simulink model "Q2_C_D_E"  (R2021a)
settings: Solver=VariableStepAuto  StartTime=0.0  StopTime=1  RelTol=1e-3
settings Model: Creator=Mohammad  LastModifiedBy=Mohammad

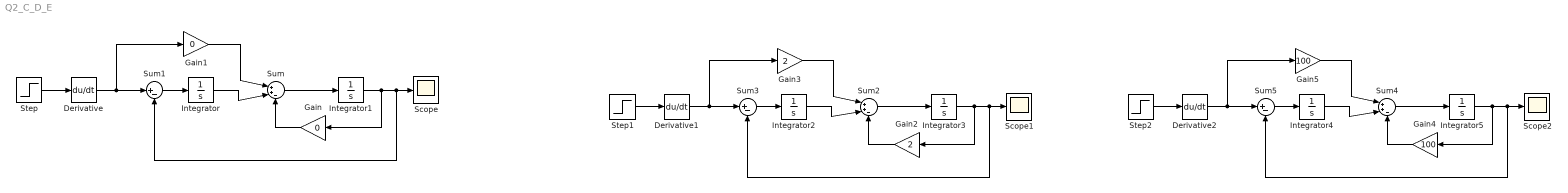
== system Q2_C_D_E ==
  Derivative : Derivative
  Derivative1 : Derivative
  Derivative2 : Derivative
  Gain : Gain  Gain=0
  Gain1 : Gain  Gain=0
  Gain2 : Gain  Gain=2
  Gain3 : Gain  Gain=2
  Gain4 : Gain  Gain=100
  Gain5 : Gain  Gain=100
  Integrator{,1..5} (6 alike) : Integrator
  Scope : Scope
  Scope1 : Scope
  Scope2 : Scope
  Step : Step  Time=0.001  SampleTime=0
  Step1 : Step  Time=0.001  SampleTime=0
  Step2 : Step  Time=0.001  SampleTime=0
  Sum : Sum  Inputs=|++-
  Sum1 : Sum  Inputs=|+-
  Sum2 : Sum  Inputs=|++-
  Sum3 : Sum  Inputs=|+-
  Sum4 : Sum  Inputs=|++-
  Sum5 : Sum  Inputs=|+-
  wires:
  Gain/1 -> Sum/3
  Gain1/1 -> Sum/1
  Integrator/1 -> Sum/2
  Sum1/1 -> Integrator/1
  Step/1 -> Derivative/1
  Derivative/1 -> Gain1/1, Sum1/1
  Sum/1 -> Integrator1/1
  Integrator1/1 -> Sum1/2, Scope/1, Gain/1
  Sum3/1 -> Integrator2/1
  Sum2/1 -> Integrator3/1
  Derivative1/1 -> Gain3/1, Sum3/1
  Gain3/1 -> Sum2/1
  Integrator2/1 -> Sum2/2
  Gain2/1 -> Sum2/3
  Step1/1 -> Derivative1/1
  Integrator3/1 -> Sum3/2, Scope1/1, Gain2/1
  Sum5/1 -> Integrator4/1
  Sum4/1 -> Integrator5/1
  Derivative2/1 -> Gain5/1, Sum5/1
  Gain5/1 -> Sum4/1
  Integrator4/1 -> Sum4/2
  Gain4/1 -> Sum4/3
  Step2/1 -> Derivative2/1
  Integrator5/1 -> Sum5/2, Scope2/1, Gain4/1
